simulink model "MVC2"  (R2019b)
settings: Solver=VariableStepAuto  StartTime=0.0  StopTime=SimulationTime  RelTol=1e-3
values from neighbouring files (symbols this model uses):
  disturbanceStrength = 0.001    [Obliczenia.m]
  RegulatedValue = 5    [Obliczenia.m]
  SampleTime = 1    [Obliczenia.m]
libraries: simulink x6
settings Model: Creator=pleka  LastModifiedBy=pleka

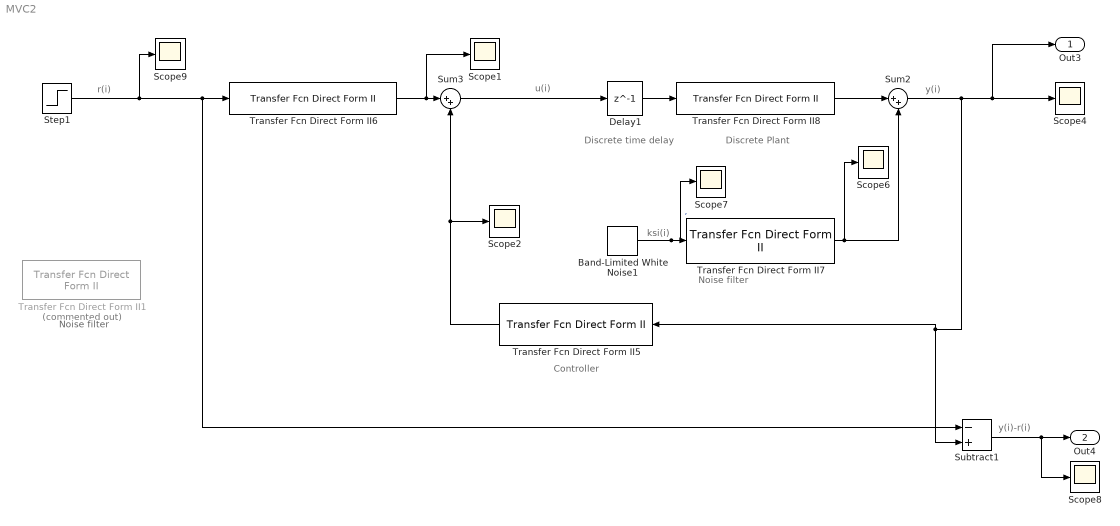
== system MVC2 ==
  note: Discrete Plant
  note: u(i)
  note: Discrete time delay
  note: Noise filter
  note: Controller
  note: r(i)
  note: y(i)-r(i)
  note: y(i)
  note: ksi(i)
  note: Noise filter
  Band-Limited White Noise1 : simulink/Sources/Band-Limited White Noise  Cov=[disturbanceStrength]  Ts=SampleTime  seed=[23341]
  Delay1 : Delay  DelayLength=1
  Scope{1..2,4,6..9} (7 alike) : Scope
  Step1 : Step  After=RegulatedValue  SampleTime=SampleTime
  Subtract1 : Sum  Inputs=-+
  Sum2 : Sum  Inputs=|++
  Sum3 : Sum  Inputs=|++
  Transfer Fcn Direct Form II1 : simulink/Additional Math & Discrete/Additional Discrete/Transfer Fcn Direct Form II  Commented=on  NumCoefVec=[1 -0.16 0.0064]  DenCoefVec=[0.96 0.2088]  vinit=0.0  DoSatur=off
      settings: SourceProductName=Simulink  SourceProductBaseCode=SL
  Transfer Fcn Direct Form II5 : simulink/Additional Math & Discrete/Additional Discrete/Transfer Fcn Direct Form II  NumCoefVec=[-2.4 1 -0.04]  DenCoefVec=[-0.4 -0.24]  vinit=0.0  DoSatur=off
      settings: SourceProductName=Simulink  SourceProductBaseCode=SL
  Transfer Fcn Direct Form II6 : simulink/Additional Math & Discrete/Additional Discrete/Transfer Fcn Direct Form II  NumCoefVec=[2 0 0]  DenCoefVec=[-0.4 -0.24]  vinit=0.0  DoSatur=off
      settings: SourceProductName=Simulink  SourceProductBaseCode=SL
  Transfer Fcn Direct Form II7 : simulink/Additional Math & Discrete/Additional Discrete/Transfer Fcn Direct Form II  NumCoefVec=[1 0 0 0]  DenCoefVec=[-1.2 0.5 -0.02]  vinit=0.0  DoSatur=off
      settings: SourceProductName=Simulink  SourceProductBaseCode=SL
  Transfer Fcn Direct Form II8 : simulink/Additional Math & Discrete/Additional Discrete/Transfer Fcn Direct Form II  NumCoefVec=[0.5 -0.2 -0.12 0]  DenCoefVec=[-1.2 0.5 -0.02]  vinit=0.0  DoSatur=off
      settings: SourceProductName=Simulink  SourceProductBaseCode=SL
  Out3 : Outport
  Out4 : Outport  Port=2
  wires:
  Step1/1 -> Transfer Fcn Direct Form II6/1, Subtract1/1, Scope9/1
  Sum3/1 -> Delay1/1
  Transfer Fcn Direct Form II7/1 -> Scope6/1, Sum2/2
  Transfer Fcn Direct Form II6/1 -> Scope1/1, Sum3/1
  Sum2/1 -> Transfer Fcn Direct Form II5/1, Subtract1/2, Out3/1, Scope4/1
  Band-Limited White Noise1/1 -> Scope7/1, Transfer Fcn Direct Form II7/1  ","
  Transfer Fcn Direct Form II5/1 -> Scope2/1, Sum3/2
  Subtract1/1 -> Scope8/1, Out4/1
  Transfer Fcn Direct Form II8/1 -> Sum2/1
  Delay1/1 -> Transfer Fcn Direct Form II8/1
